simulink model "testinput3"  (Simulink 3.00)
settings: Solver=FixedStepDiscrete  StartTime=0.0  StopTime=60.0  FixedStep=0.02  RelTol=1e-3
libraries: simulink3 x2
settings Model: LastModifiedBy=hkg

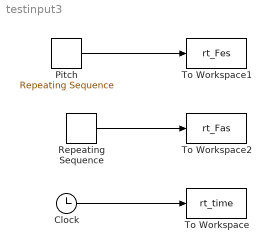
== system testinput3 ==
  Clock : Clock
      settings: DisplayTime=off  Decimation=10
  Pitch : simulink3/Sources/Repeating Sequence  rep_seq_t=[0 0.6 99 100]  rep_seq_y=[0 80 80 0]
  Repeating Sequence : simulink3/Sources/Repeating Sequence  rep_seq_t=[0 0.01 0.8 0.81 100]  rep_seq_y=[0 60 60 0 0]
  To Workspace : ToWorkspace  VariableName=rt_time  SampleTime=-1  SaveFormat=Matrix
  To Workspace1 : ToWorkspace  VariableName=rt_Fes  SampleTime=-1  SaveFormat=Matrix
  To Workspace2 : ToWorkspace  VariableName=rt_Fas  SampleTime=-1  SaveFormat=Matrix
  wires:
  Clock/1 -> To Workspace/1
  Pitch/1 -> To Workspace1/1
  Repeating Sequence/1 -> To Workspace2/1
